simulink model "swing_equation_model_general"  (R2014a)
settings: Solver=ode23t  StartTime=0.0  StopTime=1.5  RelTol=1e-3
settings Model: Creator=Divya M  LastModifiedBy=Divya M

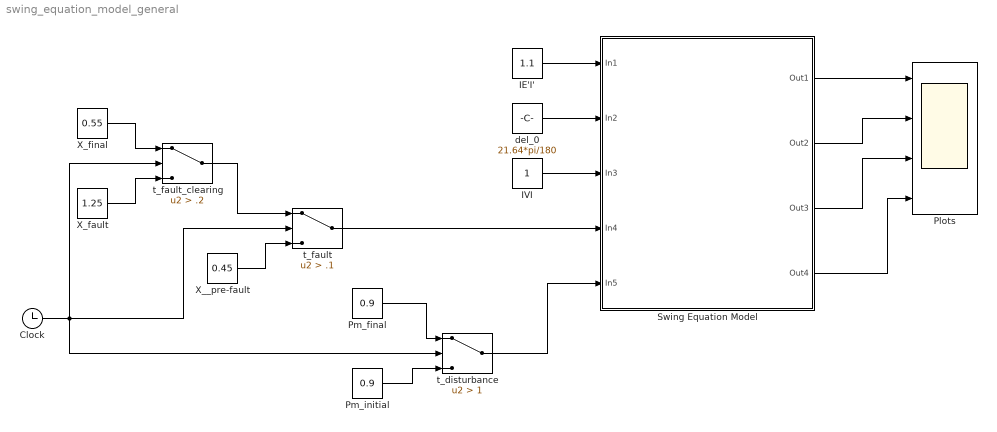
== system swing_equation_model_general ==
  Clock : Clock
  IE'I' : Constant  Value=1.1
  IVI : Constant
  Plots : Scope  NumInputPorts=4
      settings: YMin=-0.3~-1000~-10~20  YMax=0.3~1000~10~35  SaveName=ScopeData2
  Pm_final : Constant  Value=0.9
  Pm_initial : Constant  Value=0.9
  Swing Equation Model : Subsystem
  X__pre-fault : Constant  Value=0.45
  X_fault : Constant  Value=1.25
  X_final : Constant  Value=0.55
  del_0 : Constant  Value=21.64*pi/180
  t_disturbance : Switch  Criteria=u2 > Threshold  Threshold=1
  t_fault : Switch  Criteria=u2 > Threshold  Threshold=.1
  t_fault_clearing : Switch  Criteria=u2 > Threshold  Threshold=.2
  wires:
  X_final/1 -> t_fault_clearing/1
  X_fault/1 -> t_fault_clearing/3
  t_fault_clearing/1 -> t_fault/1
  Clock/1 -> t_fault_clearing/2, t_fault/2, t_disturbance/2
  X__pre-fault/1 -> t_fault/3
  IE'I'/1 -> Swing Equation Model/1(In1)
  del_0/1 -> Swing Equation Model/2(In2)
  IVI/1 -> Swing Equation Model/3(In3)
  t_fault/1 -> Swing Equation Model/4(In4)
  Pm_initial/1 -> t_disturbance/3
  Pm_final/1 -> t_disturbance/1
  t_disturbance/1 -> Swing Equation Model/5(In5)
  Swing Equation Model/1(Out1) -> Plots/1
  Swing Equation Model/2(Out2) -> Plots/2
  Swing Equation Model/3(Out3) -> Plots/3
  Swing Equation Model/4(Out4) -> Plots/4

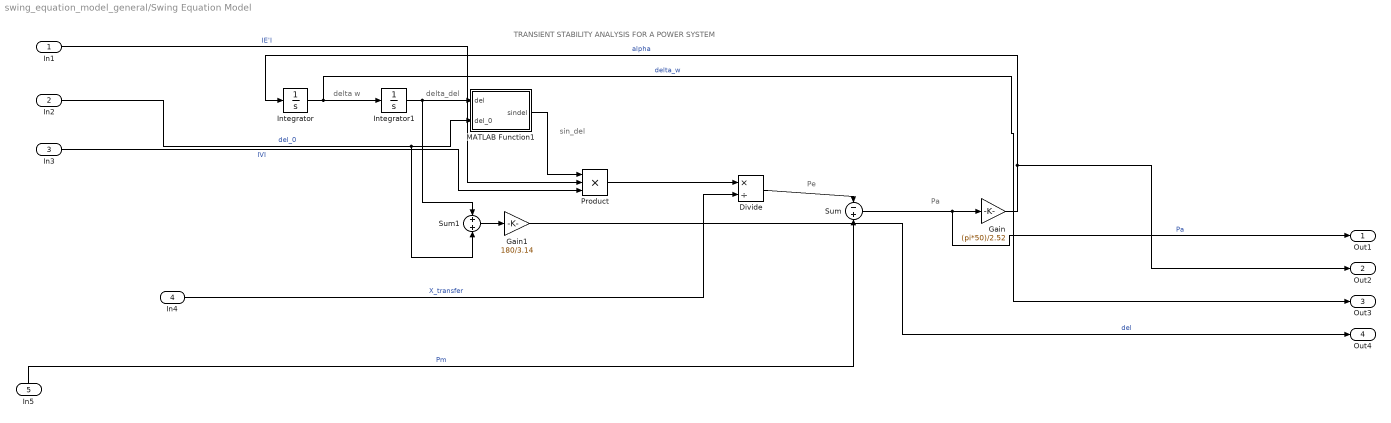
== system swing_equation_model_general/Swing Equation Model ==
  note: Pa
  note: Pe
  note: sin_del
  note: delta_del
  note: delta w
  note: TRANSIENT STABILITY ANALYSIS FOR A POWER SYSTEM
  In1 : Inport
  In2 : Inport  Port=2
  In3 : Inport  Port=3
  In4 : Inport  Port=4
  In5 : Inport  Port=5
  Divide : Product  Inputs=*/
  Gain : Gain  Gain=(pi*50)/2.52
  Gain1 : Gain  Gain=180/3.14
  Integrator : Integrator
  Integrator1 : Integrator
  MATLAB Function1 : MATLAB Function  TreatAsAtomicUnit=on
  Product : Product  Inputs=3
  Sum : Sum  Inputs=-+
  Sum1 : Sum
  Out1 : Outport
  Out2 : Outport  Port=2
  Out3 : Outport  Port=3
  Out4 : Outport  Port=4
  wires:
  MATLAB Function1/1(sindel) -> Product/1
  In2/1 -> MATLAB Function1/2(del_0), Sum1/2  "del_0"
  Integrator1/1 -> Sum1/1, MATLAB Function1/1(del)
  In4/1 -> Divide/2  "X_transfer"
  Divide/1 -> Sum/1
  Product/1 -> Divide/1
  Integrator/1 -> Out3/1, Integrator1/1  "delta_w"
  Sum/1 -> Out1/1, Gain/1  "Pa"
  In5/1 -> Sum/2  "Pm"
  Gain/1 -> Out2/1, Integrator/1  "alpha"
  In3/1 -> Product/3  "IVI"
  In1/1 -> Product/2  "IE'I"
  Sum1/1 -> Gain1/1
  Gain1/1 -> Out4/1  "del"

== matlab function swing_equation_model_general/Swing Equation Model/MATLAB Function1 ==
  data: del input; sindel output; del_0 input
%function y = fcn(u)
function sindel=fcn(del,del_0)
%del0=21.64*pi/180;
del1=del_0+del;
sindel= sin(del1);


%y = u;
